simulink model "hevPem"  (R2016b)
settings: Solver=FixedStepAuto  StartTime=0.0  StopTime=100  RelTol=1e-3
undefined symbols (not defined in the file or in its folder): h, w_em_upper
settings Model: Creator=Niklas  LastModifiedBy=Niklas
settings DataIOCC: SaveTime=off

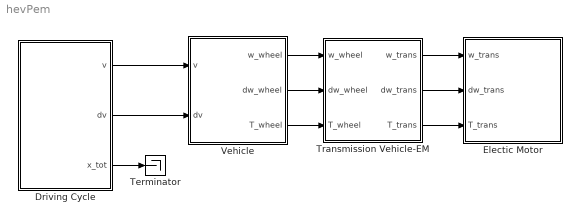
== system hevPem ==
  Driving Cycle : Subsystem  mask{Ts=1}
      mask prompts: Ts "Step size [s]"
      mask init:
      | init_drive_cycle
  Electic Motor : Subsystem  mask{theta_em=1}
      mask prompts: theta_em "Motor Ineratia [kg*m^2]"
      mask init:
      | init_EM
  Terminator : Terminator
  Transmission Vehicle-EM : Subsystem  mask{gear_ratio=0.707, eta_gb=0.975, P_gb0=0, w_wheel_min=1}
      mask prompts: gear_ratio "Gear Ratio"; eta_gb "Efficiency"; P_gb0 "Idling losses (friction) [W]"; w_wheel_min "Minimum wheel speed beyond which losses are generated [rad/s]"
      mask init:
      | init_transmission;
  Vehicle : Subsystem  mask{r_wheel=0.82, R0=554.9, R1=20.3, R2=3.56}
      mask prompts: r_wheel "Wheel Radius [m]"; R0 "Running Resistance R0 [N]"; R1 "Running Resistance R1 [N/(m/s)]"; R2 "Running Resistance R2 [N/(m/s)^2]"
      mask init:
      | init_vehicle
  wires:
  Transmission Vehicle-EM/1(w_trans) -> Electic Motor/1(w_trans)
  Transmission Vehicle-EM/2(dw_trans) -> Electic Motor/2(dw_trans)
  Transmission Vehicle-EM/3(T_trans) -> Electic Motor/3(T_trans)
  Vehicle/1(w_wheel) -> Transmission Vehicle-EM/1(w_wheel)
  Vehicle/2(dw_wheel) -> Transmission Vehicle-EM/2(dw_wheel)
  Vehicle/3(T_wheel) -> Transmission Vehicle-EM/3(T_wheel)
  Driving Cycle/1(v) -> Vehicle/1(v)
  Driving Cycle/2(dv) -> Vehicle/2(dv)
  Driving Cycle/3(x_tot) -> Terminator/1

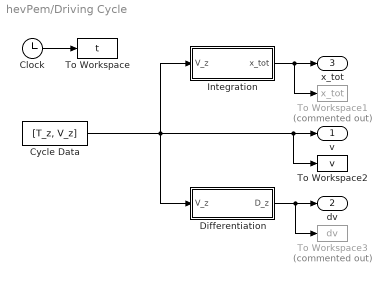
== system hevPem/Driving Cycle ==
  Clock : Clock
  Cycle Data : FromWorkspace  VariableName=[T_z, V_z]  SampleTime=h
  Differentiation : Subsystem
  Integration : Subsystem
  To Workspace : ToWorkspace  VariableName=t  SampleTime=h
  To Workspace1 : ToWorkspace  Commented=on  VariableName=x_tot  SampleTime=-1
  To Workspace2 : ToWorkspace  VariableName=v  SampleTime=-1
  To Workspace3 : ToWorkspace  Commented=on  VariableName=dv  SampleTime=-1
  v : Outport
  dv : Outport  Port=2
  x_tot : Outport  Port=3
  wires:
  Clock/1 -> To Workspace/1
  Cycle Data/1 -> Differentiation/1(V_z), Integration/1(V_z), To Workspace2/1, v/1
  Integration/1(x_tot) -> To Workspace1/1, x_tot/1
  Differentiation/1(D_z) -> To Workspace3/1, dv/1

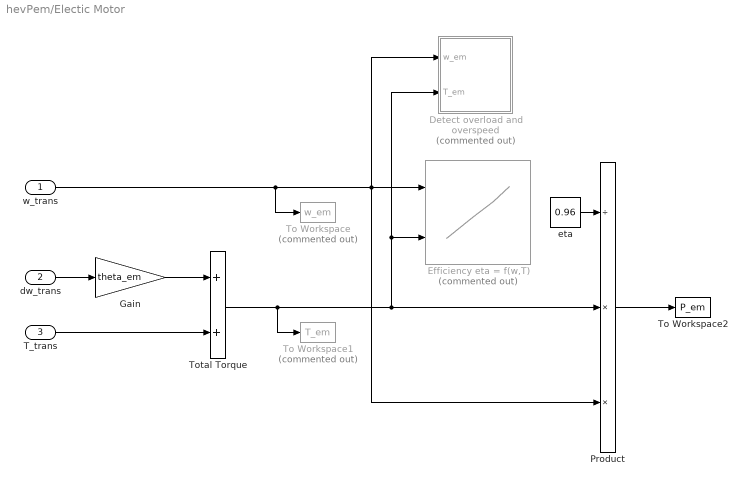
== system hevPem/Electic Motor ==
  w_trans : Inport
  dw_trans : Inport  Port=2
  T_trans : Inport  Port=3
  Detect overload and overspeed : Subsystem  Commented=on
  Efficiency eta = f(w,T) : Lookup_n-D  Commented=on  BreakpointsForDimension1=[1:3]  BreakpointsForDimension2=[1:3]  InternalRulePriority=Speed  RndMeth=Simplest  InputSameDT=on
  Gain : Gain  Gain=theta_em
  Product : Product  Inputs=/**
  To Workspace : ToWorkspace  Commented=on  VariableName=w_em  SampleTime=-1
  To Workspace1 : ToWorkspace  Commented=on  VariableName=T_em  SampleTime=-1
  To Workspace2 : ToWorkspace  VariableName=P_em  SampleTime=-1
  Total Torque : Sum
  eta : Constant  Value=0.96
  wires:
  Product/1 -> To Workspace2/1
  dw_trans/1 -> Gain/1
  Gain/1 -> Total Torque/1
  T_trans/1 -> Total Torque/2
  Total Torque/1 -> To Workspace1/1, Efficiency eta = f(w,T)/2, Detect overload and overspeed/2(T_em), Product/2
  w_trans/1 -> To Workspace/1, Product/3, Detect overload and overspeed/1(w_em), Efficiency eta = f(w,T)/1
  eta/1 -> Product/1

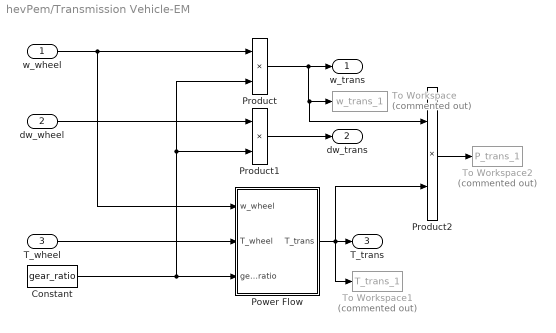
== system hevPem/Transmission Vehicle-EM ==
  w_wheel : Inport
  dw_wheel : Inport  Port=2
  T_wheel : Inport  Port=3
  Constant : Constant  Value=gear_ratio
  Power Flow : Subsystem
  Product : Product
  Product1 : Product
  Product2 : Product
  To Workspace : ToWorkspace  Commented=on  VariableName=w_trans_1  SampleTime=-1
  To Workspace1 : ToWorkspace  Commented=on  VariableName=T_trans_1  SampleTime=-1
  To Workspace2 : ToWorkspace  Commented=on  VariableName=P_trans_1  SampleTime=-1
  w_trans : Outport
  dw_trans : Outport  Port=2
  T_trans : Outport  Port=3
  wires:
  w_wheel/1 -> Product/1, Power Flow/1(w_wheel)
  dw_wheel/1 -> Product1/1
  Product/1 -> Product2/1, To Workspace/1, w_trans/1
  Power Flow/1(T_trans) -> To Workspace1/1, Product2/2, T_trans/1
  Product1/1 -> dw_trans/1
  T_wheel/1 -> Power Flow/2(T_wheel)
  Constant/1 -> Product/2, Product1/2, Power Flow/3(gear_ratio)
  Product2/1 -> To Workspace2/1

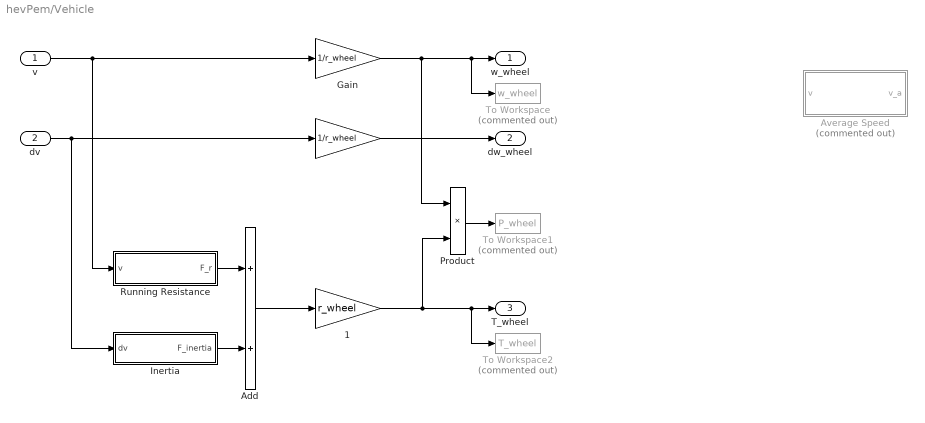
== system hevPem/Vehicle ==
  v : Inport
  dv : Inport  Port=2
  " " : Gain  Gain=1/r_wheel
  " 1" : Gain  Gain=r_wheel
  Add : Sum
  Average Speed : Subsystem  Commented=on
  Gain : Gain  Gain=1/r_wheel
  Inertia : Subsystem
  Product : Product
  Running Resistance : Subsystem
  To Workspace : ToWorkspace  Commented=on  VariableName=w_wheel  SampleTime=-1
  To Workspace1 : ToWorkspace  Commented=on  VariableName=P_wheel  SampleTime=-1
  To Workspace2 : ToWorkspace  Commented=on  VariableName=T_wheel  SampleTime=-1
  w_wheel : Outport
  dw_wheel : Outport  Port=2
  T_wheel : Outport  Port=3
  wires:
  Gain/1 -> To Workspace/1, w_wheel/1, Product/1
  " "/1 -> dw_wheel/1
  dv/1 -> Inertia/1(dv), " "/1
  " 1"/1 -> To Workspace2/1, T_wheel/1, Product/2
  Product/1 -> To Workspace1/1
  v/1 -> Gain/1, Running Resistance/1(v)
  Add/1 -> " 1"/1
  Inertia/1(F_inertia) -> Add/2
  Running Resistance/1(F_r) -> Add/1

== system hevPem/Driving Cycle/Differentiation ==
  V_z : Inport
  Add : Sum  Inputs=+-
  Unit Delay : UnitDelay  SampleTime=-1
  D_z : Outport
  wires:
  Unit Delay/1 -> Add/2
  V_z/1 -> Unit Delay/1, Add/1
  Add/1 -> D_z/1

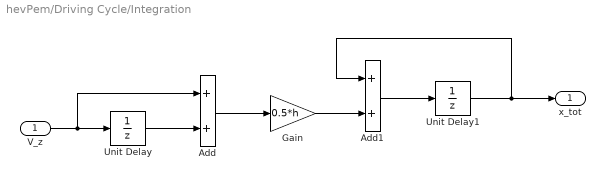
== system hevPem/Driving Cycle/Integration ==
  V_z : Inport
  Add : Sum
  Add1 : Sum
  Gain : Gain  Gain=0.5*h
  Unit Delay : UnitDelay  SampleTime=-1
  Unit Delay1 : UnitDelay  SampleTime=-1
  x_tot : Outport
  wires:
  Unit Delay/1 -> Add/2
  V_z/1 -> Add/1, Unit Delay/1
  Add/1 -> Gain/1
  Gain/1 -> Add1/2
  Add1/1 -> Unit Delay1/1
  Unit Delay1/1 -> x_tot/1, Add1/1

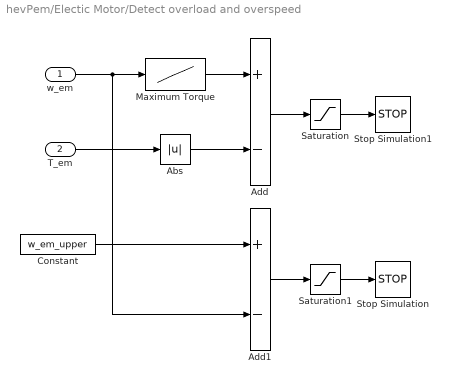
== system hevPem/Electic Motor/Detect overload and overspeed ==
  w_em : Inport
  T_em : Inport  Port=2
  Abs : Abs
  Add : Sum  Inputs=+-
  Add1 : Sum  Inputs=+-
  Constant : Constant  Value=w_em_upper
  Maximum Torque : Lookup_n-D  NumberOfTableDimensions=1  BreakpointsForDimension1=[-5:5]  Table=tanh([-5:5])  InternalRulePriority=Speed  RndMeth=Simplest  InputSameDT=on
  Saturation : Saturate  UpperLimit=0  LowerLimit=-inf
  Saturation1 : Saturate  UpperLimit=0  LowerLimit=-inf
  Stop Simulation : Stop
  Stop Simulation1 : Stop
  wires:
  w_em/1 -> Add1/2, Maximum Torque/1
  T_em/1 -> Abs/1
  Maximum Torque/1 -> Add/1
  Abs/1 -> Add/2
  Add/1 -> Saturation/1
  Saturation/1 -> Stop Simulation1/1
  Constant/1 -> Add1/1
  Add1/1 -> Saturation1/1
  Saturation1/1 -> Stop Simulation/1

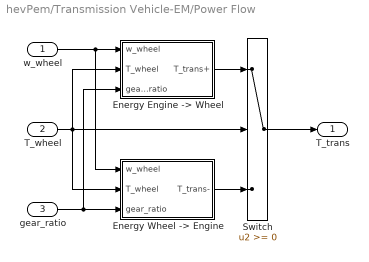
== system hevPem/Transmission Vehicle-EM/Power Flow ==
  w_wheel : Inport
  T_wheel : Inport  Port=2
  gear_ratio : Inport  Port=3
  "Energy Engine -> Wheel" : Subsystem
  "Energy Wheel -> Engine" : Subsystem
  Switch : Switch
  T_trans : Outport
  wires:
  T_wheel/1 -> "Energy Wheel -> Engine"/2(T_wheel), "Energy Engine -> Wheel"/2(T_wheel), Switch/2
  Switch/1 -> T_trans/1
  "Energy Wheel -> Engine"/1(T_trans-) -> Switch/3
  "Energy Engine -> Wheel"/1(T_trans+) -> Switch/1
  gear_ratio/1 -> "Energy Wheel -> Engine"/3(gear_ratio), "Energy Engine -> Wheel"/3(gear_ratio)
  w_wheel/1 -> "Energy Wheel -> Engine"/1(w_wheel), "Energy Engine -> Wheel"/1(w_wheel)

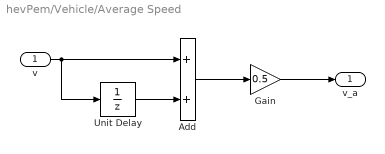
== system hevPem/Vehicle/Average Speed ==
  v : Inport
  Add : Sum
  Gain : Gain  Gain=0.5
  Unit Delay : UnitDelay  SampleTime=-1
  v_a : Outport
  wires:
  v/1 -> Unit Delay/1, Add/1
  Unit Delay/1 -> Add/2
  Add/1 -> Gain/1
  Gain/1 -> v_a/1

== system hevPem/Vehicle/Inertia ==
  dv : Inport
  Inertia : Fcn  Expr=39600*(1.08)*u/h
  F_inertia : Outport
  wires:
  dv/1 -> Inertia/1
  Inertia/1 -> F_inertia/1

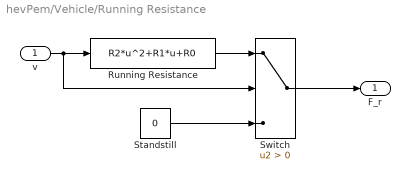
== system hevPem/Vehicle/Running Resistance ==
  v : Inport
  Running Resistance : Fcn  Expr=R2*u^2+R1*u+R0
  Standstill : Constant  Value=0
  Switch : Switch  Criteria=u2 > Threshold
  F_r : Outport
  wires:
  Running Resistance/1 -> Switch/1
  v/1 -> Switch/2, Running Resistance/1
  Switch/1 -> F_r/1
  Standstill/1 -> Switch/3

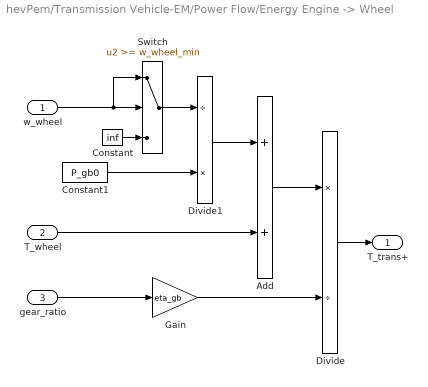
== system hevPem/Transmission Vehicle-EM/Power Flow/Energy Engine -> Wheel ==
  w_wheel : Inport
  T_wheel : Inport  Port=2
  gear_ratio : Inport  Port=3
  Add : Sum
  Constant : Constant  Value=inf
  Constant1 : Constant  Value=P_gb0
  Divide : Product  Inputs=*/
  Divide1 : Product  Inputs=/*
  Gain : Gain  Gain=eta_gb
  Switch : Switch  Threshold=w_wheel_min
  T_trans+ : Outport
  wires:
  Divide/1 -> T_trans+/1
  Add/1 -> Divide/1
  Divide1/1 -> Add/1
  Switch/1 -> Divide1/1
  w_wheel/1 -> Switch/1, Switch/2
  Constant/1 -> Switch/3
  T_wheel/1 -> Add/2
  Constant1/1 -> Divide1/2
  Gain/1 -> Divide/2
  gear_ratio/1 -> Gain/1

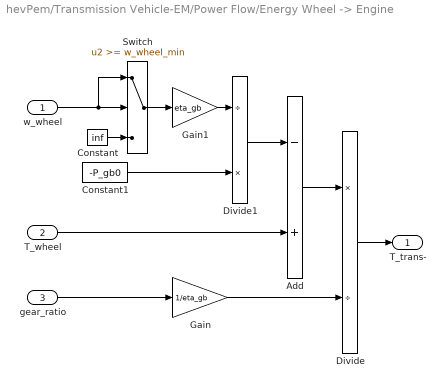
== system hevPem/Transmission Vehicle-EM/Power Flow/Energy Wheel -> Engine ==
  w_wheel : Inport
  T_wheel : Inport  Port=2
  gear_ratio : Inport  Port=3
  Add : Sum  Inputs=-+
  Constant : Constant  Value=inf
  Constant1 : Constant  Value=-P_gb0
  Divide : Product  Inputs=*/
  Divide1 : Product  Inputs=/*
  Gain : Gain  Gain=1/eta_gb
  Gain1 : Gain  Gain=eta_gb
  Switch : Switch  Threshold=w_wheel_min
  T_trans- : Outport
  wires:
  Divide/1 -> T_trans-/1
  Add/1 -> Divide/1
  Divide1/1 -> Add/1
  w_wheel/1 -> Switch/1, Switch/2
  Constant/1 -> Switch/3
  T_wheel/1 -> Add/2
  Constant1/1 -> Divide1/2
  Gain/1 -> Divide/2
  gear_ratio/1 -> Gain/1
  Switch/1 -> Gain1/1
  Gain1/1 -> Divide1/1
